simulink library "inter_fir_lib"  (Simulink 7.3)
settings: Solver=ode45  SolverMode=SingleTasking  StartTime=0.0  StopTime=10.0  RelTol=1e-3
libraries: xbsIndex_r4 x40, casper_library x2
settings Model: Creator=rprimian  LastModifiedBy=rprimian

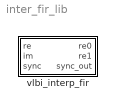
== system inter_fir_lib ==
  vlbi_interp_fir : Subsystem  mask{tap_delay=16, n_bits=18, add_latency=2, mult_latency=3, bram_latency=2}
      mask prompts: tap_delay "Delay between Taps"; n_bits "Bit Width"; add_latency "Add Latency"; mult_latency "Mult Latency"; bram_latency "BRAM Latency"
      mask init:
      | for i=0:4,
      |     x = pi*(2*i+1)/2;
      |     coeff(i+1) = sin(x)/x;
      | end
      | coeff = coeff / (2*sum(coeff));

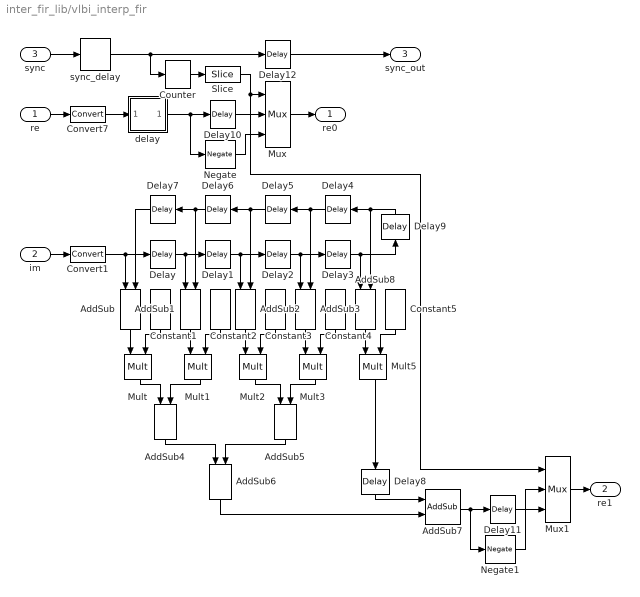
== system inter_fir_lib/vlbi_interp_fir ==
  re : Inport  OutDataType=sfix(16)  OutScaling=2^0
  im : Inport  Port=2  OutDataType=sfix(16)  OutScaling=2^0
  sync : Inport  Port=3  OutDataType=sfix(16)  OutScaling=2^0
  AddSub{,1,3..8} (8 alike) : xbsIndex_r4/AddSub  mode=Addition  use_carryin=off  use_carryout=off  en=off  latency=add_latency  precision=Full  arith_type=Unsigned  n_bits=8  bin_pt=2  quantization=Truncate  overflow=Wrap  dbl_ovrd=off  use_behavioral_HDL=on  hw_selection=Fabric  pipelined=on  use_rpm=off  block_type=addsub
      settings: xl_area=[0, 0, 0, 0, 0, 0, 0]  block_version=11.3
  AddSub2 : xbsIndex_r4/AddSub  mode=Addition  use_carryin=off  use_carryout=off  en=off  latency=add_latency  precision=Full  arith_type=Unsigned  n_bits=8  bin_pt=2  quantization=Truncate  overflow=Wrap  dbl_ovrd=off  use_behavioral_HDL=on  hw_selection=Fabric  pipelined=off  use_rpm=on  block_type=addsub
      settings: xl_area=[0, 0, 0, 0, 0, 0, 0]  block_version=11.3
  Constant1 : xbsIndex_r4/Constant  arith_type=Signed (2's comp)  const=coeff(5)  n_bits=n_bits  bin_pt=n_bits - 1  explicit_period=on  period=1  equ=P=C  opselect=C  inp2=PCIN>>17  opr=+  inp1=P  carry=CIN  dbl_ovrd=off  block_type=constant
      settings: block_version=11.3
  Constant2 : xbsIndex_r4/Constant  arith_type=Signed (2's comp)  const=coeff(4)  n_bits=n_bits  bin_pt=n_bits-1  explicit_period=on  period=1  equ=P=C  opselect=C  inp2=PCIN>>17  opr=+  inp1=P  carry=CIN  dbl_ovrd=off  block_type=constant
      settings: block_version=11.3
  Constant3 : xbsIndex_r4/Constant  arith_type=Signed (2's comp)  const=coeff(3)  n_bits=n_bits  bin_pt=n_bits-1  explicit_period=on  period=1  equ=P=C  opselect=C  inp2=PCIN>>17  opr=+  inp1=P  carry=CIN  dbl_ovrd=off  block_type=constant
      settings: block_version=11.3
  Constant4 : xbsIndex_r4/Constant  arith_type=Signed (2's comp)  const=coeff(2)  n_bits=n_bits  bin_pt=n_bits-1  explicit_period=on  period=1  equ=P=C  opselect=C  inp2=PCIN>>17  opr=+  inp1=P  carry=CIN  dbl_ovrd=off  block_type=constant
      settings: block_version=11.3
  Constant5 : xbsIndex_r4/Constant  arith_type=Signed (2's comp)  const=coeff(1)  n_bits=n_bits  bin_pt=n_bits-1  explicit_period=on  period=1  equ=P=C  opselect=C  inp2=PCIN>>17  opr=+  inp1=P  carry=CIN  dbl_ovrd=off  block_type=constant
      settings: block_version=11.3
  Convert1 : xbsIndex_r4/Convert  arith_type="Signed  (2's comp)"  n_bits=n_bits - 1  bin_pt=n_bits - 2  quantization=Truncate  overflow=Wrap  latency=add_latency  dbl_ovrd=off  pipeline=on  block_type=convert
      settings: xl_area=[0, 0, 0, 0, 0, 0, 0]  block_version=11.3
  Convert7 : xbsIndex_r4/Convert  arith_type="Signed  (2's comp)"  n_bits=n_bits  bin_pt=n_bits - 1  quantization=Truncate  overflow=Wrap  latency=add_latency  dbl_ovrd=off  pipeline=on  block_type=convert
      settings: xl_area=[0, 0, 0, 0, 0, 0, 0]  block_version=11.3
  Counter : xbsIndex_r4/Counter  cnt_type=Free Running  cnt_to=Inf  operation=Up  start_count=0  cnt_by_val=1  arith_type=Unsigned  n_bits=log2(tap_delay) + 1  bin_pt=0  load_pin=off  rst=on  en=off  explicit_period=off  period=1  dbl_ovrd=off  use_behavioral_HDL=off  implementation=Fabric  use_rpm=on  block_type=counter
      settings: xl_area=[0, 0, 0, 0, 0, 0, 0]  block_version=11.3
  Delay{,1..7,9} (9 alike) : xbsIndex_r4/Delay  en=off  latency=tap_delay  dbl_ovrd=off  reg_retiming=off  block_type=delay
      settings: xl_area=[0, 0, 0, 0, 0, 0, 0]  block_version=11.3
  Delay10 : xbsIndex_r4/Delay  en=off  latency=1  dbl_ovrd=off  reg_retiming=off  block_type=delay
      settings: xl_area=[0, 0, 0, 0, 0, 0, 0]  block_version=11.3
  Delay11 : xbsIndex_r4/Delay  en=off  latency=1  dbl_ovrd=off  reg_retiming=off  block_type=delay
      settings: xl_area=[0, 0, 0, 0, 0, 0, 0]  block_version=11.3
  Delay12 : xbsIndex_r4/Delay  en=off  latency=2  dbl_ovrd=off  reg_retiming=off  block_type=delay
      settings: xl_area=[0, 0, 0, 0, 0, 0, 0]  block_version=11.3
  Delay8 : xbsIndex_r4/Delay  en=off  latency=2 * add_latency  dbl_ovrd=off  reg_retiming=off  block_type=delay
      settings: xl_area=[0, 0, 0, 0, 0, 0, 0]  block_version=11.3
  Mult{,1..3,5} (5 alike) : xbsIndex_r4/Mult  precision=Full  arith_type="Signed  (2's comp)"  n_bits=8  bin_pt=2  quantization=Truncate  overflow=Wrap  en=off  latency=mult_latency  dbl_ovrd=off  use_behavioral_HDL=off  opt=Speed  use_embedded=on  optimum_pipeline=off  pipeline=on  use_rpm=off  placement_style=Rectangular shape  block_type=mult
      settings: xl_area=[0, 0, 0, 0, 0, 0, 0]  block_version=11.3
  Mux : xbsIndex_r4/Mux  inputs=2  en=off  latency=1  precision=Full  arith_type="Signed  (2's comp)"  n_bits=8  bin_pt=2  quantization=Truncate  overflow=Wrap  dbl_ovrd=off  block_type=mux
      settings: xl_area=[0, 0, 0, 0, 0, 0, 0]  block_version=11.3
  Mux1 : xbsIndex_r4/Mux  inputs=2  en=off  latency=1  precision=Full  arith_type="Signed  (2's comp)"  n_bits=8  bin_pt=2  quantization=Truncate  overflow=Wrap  dbl_ovrd=off  block_type=mux
      settings: xl_area=[0, 0, 0, 0, 0, 0, 0]  block_version=11.3
  Negate : xbsIndex_r4/Negate  precision=Full  arith_type=Unsigned  n_bits=8  bin_pt=2  quantization=Truncate  overflow=Wrap  en=off  latency=1  dbl_ovrd=off  block_type=negate
      settings: xl_area=[0, 0, 0, 0, 0, 0, 0]  block_version=11.3
  Negate1 : xbsIndex_r4/Negate  precision=Full  arith_type=Unsigned  n_bits=8  bin_pt=2  quantization=Truncate  overflow=Wrap  en=off  latency=1  dbl_ovrd=off  block_type=negate
      settings: xl_area=[0, 0, 0, 0, 0, 0, 0]  block_version=11.3
  Slice : xbsIndex_r4/Slice  nbits=1  boolean_output=off  mode=Upper Bit Location + Width  bit1=0  base1=MSB of Input  bit0=0  base0=LSB of Input  dbl_ovrd=off  block_type=slice
      settings: block_version=11.3
  delay : Subsystem  BlockChoice=delay_bram
      link override delay_bram: DelayLen=4 * add_latency + mult_latency + 5 * tap_delay  bram_latency=bram_latency
      link override delay_bram/Constant2: equ=P=C
      link override delay_slr: DelayLen=4 * add_latency + mult_latency + 5 * tap_delay
      settings: AttributesFormatString=%<BlockChoice>  MemberBlocks=delay_bram,delay_slr
  sync_delay : casper_library/Delays/sync_delay  DelayLen=5 * add_latency + mult_latency + 5 * tap_delay
  re0 : Outport  OutDataType=sfix(16)  OutScaling=2^0
  re1 : Outport  Port=2  OutDataType=sfix(16)  OutScaling=2^0
  sync_out : Outport  Port=3  OutDataType=sfix(16)  OutScaling=2^0
  wires:
  Constant4/1 -> Mult3/2
  Constant3/1 -> Mult2/2
  Constant2/1 -> Mult1/2
  Constant1/1 -> Mult/2
  AddSub6/1 -> AddSub7/2
  AddSub5/1 -> AddSub6/2
  AddSub4/1 -> AddSub6/1
  Mult3/1 -> AddSub5/2
  Mult2/1 -> AddSub5/1
  Mult1/1 -> AddSub4/2
  Mult/1 -> AddSub4/1
  AddSub3/1 -> Mult3/1
  AddSub2/1 -> Mult2/1
  AddSub1/1 -> Mult1/1
  AddSub/1 -> Mult/1
  Delay5/1 -> AddSub2/2, Delay6/1
  Delay4/1 -> AddSub3/2, Delay5/1
  Delay2/1 -> AddSub3/1, Delay3/1
  Delay1/1 -> AddSub2/1, Delay2/1
  Delay6/1 -> AddSub1/2, Delay7/1
  Delay/1 -> AddSub1/1, Delay1/1
  Delay7/1 -> AddSub/2
  im/1 -> Convert1/1
  Delay3/1 -> Delay9/1, AddSub8/1
  Delay9/1 -> Delay4/1, AddSub8/2
  Constant5/1 -> Mult5/2
  AddSub8/1 -> Mult5/1
  Delay8/1 -> AddSub7/1
  Mult5/1 -> Delay8/1
  sync/1 -> sync_delay/1
  re/1 -> Convert7/1
  Convert7/1 -> delay/1(In1)
  Convert1/1 -> AddSub/1, Delay/1
  delay/1(Out1) -> Delay10/1, Negate/1
  Delay10/1 -> Mux/2
  Negate/1 -> Mux/3
  AddSub7/1 -> Delay11/1, Negate1/1
  Negate1/1 -> Mux1/2
  Delay11/1 -> Mux1/3
  Mux1/1 -> re1/1
  Counter/1 -> Slice/1
  sync_delay/1 -> Counter/1, Delay12/1
  Delay12/1 -> sync_out/1
  Mux/1 -> re0/1
  Slice/1 -> Mux/1, Mux1/1

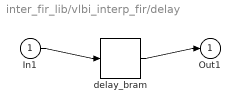
== system inter_fir_lib/vlbi_interp_fir/delay ==
  In1 : Inport  OutDataType=sfix(16)  OutScaling=2^0
  delay_bram : casper_library/Delays/delay_bram  DelayLen=4 * add_latency + mult_latency + 5 * tap_delay  bram_latency=bram_latency
  Out1 : Outport  OutDataType=sfix(16)  OutScaling=2^0
  wires:
  In1/1 -> delay_bram/1
  delay_bram/1 -> Out1/1
